simulink model "uz_pu_conversion"  (R2021a)
settings: Solver=FixedStepDiscrete  StartTime=0.0  StopTime=0.0034  RelTol=1e-3
values from neighbouring files (symbols this model uses):
  ampl = 28*sqrt(2)    [uz_pu_conversion_init.m]
  freq_Hz = 300    [uz_pu_conversion_init.m]
  I_B = sqrt(2)*I_R    [uz_pu_conversion_init.m]
  t_ADC = 1/f_ADC    (= 1e-05)    [uz_pu_conversion_init.m]
  V_B = sqrt(2/3)*V_R    [uz_pu_conversion_init.m]
  v_dc = 565    [uz_pu_conversion_init.m]
libraries: spsThreePhaseSineGeneratorLib x3, simulink x1
settings Model: DataTypeOverride=Off  Creator=micha  LastModifiedBy=micha
settings SolverCC: AlgebraicLoopSolver=TrustRegion
settings DataIOCC: LimitDataPoints=on  SaveOutput=off  SaveTime=off
settings OptimizationCC: BlockReduction=off  ConditionallyExecuteInputs=off  DefaultParameterBehavior=Inlined  LifeSpan=inf
settings DebuggingCC: AlgebraicLoopMsg=error  SingleTaskRateTransMsg=error  AllowSymbolicDim=off  StrictBusMsg=ErrorOnBusTreatedAsVector  SFUnexpectedBacktrackingDiag=warning  SFNoUnconditionalDefaultTransitionDiag=warning  SFExecutionAtInitializationDiag=none  SFMachineParentedDataDiag=warning  ArithmeticOperatorsInVariantConditions=warning
settings HardwareCC: ProdBitPerPointer=32  ProdBitPerSizeT=32  ProdBitPerPtrDiffT=32  ProdLargestAtomicFloat=None  ProdIntDivRoundTo=Undefined  ProdEndianess=Unspecified  ProdWordSize=32  ProdHWDeviceType=ASIC/FPGA->ASIC/FPGA  ProdEqTarget=off
settings SFSimCC: SimUseLocalCustomCode=off  CustomCodeUndefinedFunction=UseInterfaceOnly
settings RTWCC: RTWUseLocalCustomCode=off
settings CodeAppCC: StateflowObjectComments=on
settings GRTTargetCC: TargetLangStandard=C89/C90 (ANSI)
settings ConfigComp: CovScope=ReferencedModels  CovMetricSettings=dw  CovSaveCumulativeToWorkspaceVar=on  CovSaveSingleToWorkspaceVar=on  CovExternalEMLEnable=off  CovSFcnEnable=off

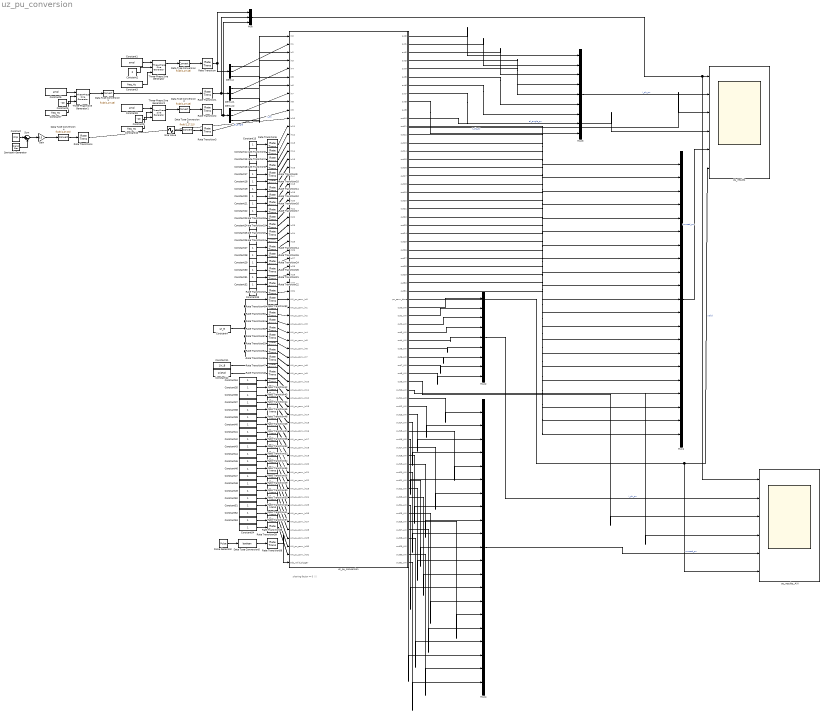
== system uz_pu_conversion ==
  note: sharing factor = 0 !!!
  Constant : Constant  Value=2*pi
  Constant1 : Constant  Value=ampl
  Constant10 : Constant  Value=freq_Hz
  Constant11 : Constant  Value=1/V_B  OutDataTypeStr=fixdt(0,18,18)
  Constant12 : Constant  Value=1/(2*pi)  OutDataTypeStr=fixdt(0,18,18)
  Constant{13..33} (21 alike) : Constant  OutDataTypeStr=fixdt(1,27,15)
  Constant2 : Constant  Value=0
  Constant3 : Constant  Value=freq_Hz
  Constant{34..54} (21 alike) : Constant  OutDataTypeStr=fixdt(0,18,18)
  Constant4 : Constant  Value=1/I_B  OutDataTypeStr=fixdt(0,18,18)
  Constant5 : Constant  Value=ampl
  Constant6 : Constant  Value=-20
  Constant7 : Constant  Value=freq_Hz
  Constant8 : Constant  Value=ampl
  Constant9 : Constant  Value=-40
  Data Type Conversion{,1..4} (5 alike) : DataTypeConversion  OutDataTypeStr=fixdt(1,27,15)
  Data Type Conversion5 : DataTypeConversion  OutDataTypeStr=boolean
  Demux : Demux  Outputs=3
  Demux1 : Demux  Outputs=3
  Demux2 : Demux  Outputs=3
  Gain : Gain  Gain=0.5
  Mux : Mux  Inputs=3
  Mux1 : Mux  Inputs=21
  Mux2 : Mux  Inputs=9
  Mux3 : Mux  Inputs=9
  Mux4 : Mux  Inputs=21
  Pulse Generator : DiscretePulseGenerator  PulseType=Time based  Period=t_ADC  PulseWidth=5
  Rate Transition{,1..58} (59 alike) : RateTransition  OutPortSampleTime=ts
  Sawtooth Generator : SignalGenerator  WaveForm=sawtooth  Amplitude=2*pi  Frequency=2*pi*freq_Hz  Units=rad/sec
  Sine Wave : Sin  Amplitude=0.03*v_dc  Bias=v_dc  Frequency=2*pi*2*9*freq_Hz  SampleTime=0
  Sum : Sum  Inputs=|+-
  Three-Phase Sine Generator : spsThreePhaseSineGeneratorLib/Three-Phase Sine Generator  Ts=10e-9
      settings: SourceProductBaseCode=PS
  Three-Phase Sine Generator1 : spsThreePhaseSineGeneratorLib/Three-Phase Sine Generator  Ts=10e-9
      settings: SourceProductBaseCode=PS
  Three-Phase Sine Generator2 : spsThreePhaseSineGeneratorLib/Three-Phase Sine Generator  Ts=10e-9
      settings: SourceProductBaseCode=PS
  pu_results : Scope  NumInputPorts=6
  pu_results_AXI : Scope  NumInputPorts=6
  uz_pu_conversion : Subsystem  TreatAsAtomicUnit=on
  wires:
  Three-Phase Sine Generator/1 -> Data Type Conversion/1
  Constant1/1 -> Three-Phase Sine Generator/1
  Constant2/1 -> Three-Phase Sine Generator/2
  Constant3/1 -> Three-Phase Sine Generator/3
  Rate Transition/1 -> Demux/1, Mux/1
  Demux/1 -> uz_pu_conversion/1(in0)
  Data Type Conversion/1 -> Rate Transition/1
  Demux/2 -> uz_pu_conversion/2(in1)
  Demux/3 -> uz_pu_conversion/3(in2)
  Constant6/1 -> Three-Phase Sine Generator1/2
  Constant7/1 -> Three-Phase Sine Generator1/3
  Data Type Conversion1/1 -> Rate Transition1/1
  Constant5/1 -> Three-Phase Sine Generator1/1
  Three-Phase Sine Generator1/1 -> Data Type Conversion1/1
  Constant4/1 -> Rate Transition56/1, Rate Transition52/1, Rate Transition49/1, Rate Transition50/1, Rate Transition51/1, Rate Transition57/1, Rate Transition53/1, Rate Transition54/1, Rate Transition55/1
  uz_pu_conversion/6(out5) -> Mux3/6
  uz_pu_conversion/5(out4) -> Mux3/5
  uz_pu_conversion/1(out0) -> Mux3/1
  uz_pu_conversion/2(out1) -> Mux3/2
  uz_pu_conversion/3(out2) -> Mux3/3
  uz_pu_conversion/4(out3) -> Mux3/4
  Mux3/1 -> pu_results/2  "i_ph_pu"
  Demux1/1 -> uz_pu_conversion/4(in3)
  Demux1/2 -> uz_pu_conversion/5(in4)
  Demux1/3 -> uz_pu_conversion/6(in5)
  Data Type Conversion2/1 -> Rate Transition2/1
  Constant8/1 -> Three-Phase Sine Generator2/1
  Three-Phase Sine Generator2/1 -> Data Type Conversion2/1
  Constant9/1 -> Three-Phase Sine Generator2/2
  Constant10/1 -> Three-Phase Sine Generator2/3
  Rate Transition2/1 -> Mux/3, Demux2/1
  Demux2/1 -> uz_pu_conversion/7(in6)
  Demux2/2 -> uz_pu_conversion/8(in7)
  Demux2/3 -> uz_pu_conversion/9(in8)
  uz_pu_conversion/7(out6) -> Mux3/7
  uz_pu_conversion/8(out7) -> Mux3/8
  uz_pu_conversion/9(out8) -> Mux3/9
  Constant11/1 -> Rate Transition47/1
  Rate Transition3/1 -> uz_pu_conversion/10(in9)  "v_dc"
  Sine Wave/1 -> Data Type Conversion3/1
  uz_pu_conversion/10(out9) -> pu_results/3  "v_dc_pu"
  Data Type Conversion3/1 -> Rate Transition3/1
  Data Type Conversion4/1 -> Rate Transition4/1
  Rate Transition4/1 -> uz_pu_conversion/11(in10)  "el_angle"
  Sawtooth Generator/1 -> Sum/2
  Constant12/1 -> Rate Transition48/1
  uz_pu_conversion/11(out10) -> pu_results/4  "el_angle_pu"
  Constant/1 -> Sum/1
  Gain/1 -> Data Type Conversion4/1
  Sum/1 -> Gain/1
  Rate Transition5/1 -> uz_pu_conversion/12(in11)
  Rate Transition6/1 -> uz_pu_conversion/13(in12)
  Rate Transition7/1 -> uz_pu_conversion/14(in13)
  Rate Transition8/1 -> uz_pu_conversion/15(in14)
  Rate Transition9/1 -> uz_pu_conversion/16(in15)
  Rate Transition10/1 -> uz_pu_conversion/17(in16)
  Rate Transition12/1 -> uz_pu_conversion/19(in18)
  Rate Transition11/1 -> uz_pu_conversion/18(in17)
  Rate Transition13/1 -> uz_pu_conversion/25(in24)
  Rate Transition16/1 -> uz_pu_conversion/20(in19)
  Rate Transition17/1 -> uz_pu_conversion/21(in20)
  Rate Transition19/1 -> uz_pu_conversion/23(in22)
  Rate Transition18/1 -> uz_pu_conversion/22(in21)
  Rate Transition20/1 -> uz_pu_conversion/24(in23)
  Rate Transition15/1 -> uz_pu_conversion/27(in26)
  Rate Transition14/1 -> uz_pu_conversion/26(in25)
  Rate Transition23/1 -> uz_pu_conversion/32(in31)
  Rate Transition22/1 -> uz_pu_conversion/31(in30)
  Rate Transition25/1 -> uz_pu_conversion/29(in28)
  Rate Transition24/1 -> uz_pu_conversion/28(in27)
  Rate Transition21/1 -> uz_pu_conversion/30(in29)
  Rate Transition34/1 -> uz_pu_conversion/54(AXI_pu_conv_in21)
  Rate Transition32/1 -> uz_pu_conversion/52(AXI_pu_conv_in19)
  Rate Transition36/1 -> uz_pu_conversion/56(AXI_pu_conv_in23)
  Rate Transition31/1 -> uz_pu_conversion/59(AXI_pu_conv_in26)
  Rate Transition43/1 -> uz_pu_conversion/45(AXI_pu_conv_in12)
  Rate Transition39/1 -> uz_pu_conversion/64(AXI_pu_conv_in31)
  Rate Transition41/1 -> uz_pu_conversion/61(AXI_pu_conv_in28)
  Rate Transition38/1 -> uz_pu_conversion/63(AXI_pu_conv_in30)
  Rate Transition30/1 -> uz_pu_conversion/58(AXI_pu_conv_in25)
  Rate Transition37/1 -> uz_pu_conversion/62(AXI_pu_conv_in29)
  Rate Transition27/1 -> uz_pu_conversion/50(AXI_pu_conv_in17)
  Rate Transition26/1 -> uz_pu_conversion/49(AXI_pu_conv_in16)
  Rate Transition40/1 -> uz_pu_conversion/60(AXI_pu_conv_in27)
  Rate Transition45/1 -> uz_pu_conversion/47(AXI_pu_conv_in14)
  Rate Transition44/1 -> uz_pu_conversion/46(AXI_pu_conv_in13)
  Rate Transition28/1 -> uz_pu_conversion/51(AXI_pu_conv_in18)
  Rate Transition35/1 -> uz_pu_conversion/55(AXI_pu_conv_in22)
  Rate Transition46/1 -> uz_pu_conversion/48(AXI_pu_conv_in15)
  Rate Transition29/1 -> uz_pu_conversion/57(AXI_pu_conv_in24)
  Rate Transition33/1 -> uz_pu_conversion/53(AXI_pu_conv_in20)
  Rate Transition42/1 -> uz_pu_conversion/44(AXI_pu_conv_in11)
  Rate Transition47/1 -> uz_pu_conversion/42(AXI_pu_conv_in9)
  Rate Transition48/1 -> uz_pu_conversion/43(AXI_pu_conv_in10)
  Rate Transition50/1 -> uz_pu_conversion/35(AXI_pu_conv_in2)
  Rate Transition49/1 -> uz_pu_conversion/34(AXI_pu_conv_in1)
  Rate Transition53/1 -> uz_pu_conversion/39(AXI_pu_conv_in6)
  Rate Transition52/1 -> uz_pu_conversion/33(AXI_pu_conv_in0)
  Rate Transition51/1 -> uz_pu_conversion/36(AXI_pu_conv_in3)
  Rate Transition54/1 -> uz_pu_conversion/40(AXI_pu_conv_in7)
  Rate Transition55/1 -> uz_pu_conversion/41(AXI_pu_conv_in8)
  Rate Transition57/1 -> uz_pu_conversion/38(AXI_pu_conv_in5)
  Rate Transition56/1 -> uz_pu_conversion/37(AXI_pu_conv_in4)
  Mux/1 -> pu_results/1, pu_results_AXI/1
  Rate Transition1/1 -> Mux/2, Demux1/1
  Constant13/1 -> Rate Transition5/1
  Constant14/1 -> Rate Transition6/1
  Constant15/1 -> Rate Transition7/1
  Constant16/1 -> Rate Transition8/1
  Constant18/1 -> Rate Transition10/1
  Constant17/1 -> Rate Transition9/1
  Constant19/1 -> Rate Transition11/1
  Constant20/1 -> Rate Transition12/1
  Constant22/1 -> Rate Transition17/1
  Constant21/1 -> Rate Transition16/1
  Constant23/1 -> Rate Transition18/1
  Constant24/1 -> Rate Transition19/1
  Constant26/1 -> Rate Transition13/1
  Constant25/1 -> Rate Transition20/1
  Constant27/1 -> Rate Transition14/1
  Constant28/1 -> Rate Transition15/1
  Constant30/1 -> Rate Transition25/1
  Constant29/1 -> Rate Transition24/1
  Constant32/1 -> Rate Transition22/1
  Constant31/1 -> Rate Transition21/1
  Constant33/1 -> Rate Transition23/1
  Constant34/1 -> Rate Transition42/1
  Constant35/1 -> Rate Transition43/1
  Constant37/1 -> Rate Transition45/1
  Constant36/1 -> Rate Transition44/1
  Constant41/1 -> Rate Transition28/1
  Constant40/1 -> Rate Transition27/1
  Constant39/1 -> Rate Transition26/1
  Constant38/1 -> Rate Transition46/1
  Constant47/1 -> Rate Transition29/1
  Constant46/1 -> Rate Transition36/1
  Constant49/1 -> Rate Transition31/1
  Constant45/1 -> Rate Transition35/1
  Constant48/1 -> Rate Transition30/1
  Constant44/1 -> Rate Transition34/1
  Constant43/1 -> Rate Transition33/1
  Constant42/1 -> Rate Transition32/1
  Constant53/1 -> Rate Transition38/1
  Constant54/1 -> Rate Transition39/1
  Constant50/1 -> Rate Transition40/1
  Constant51/1 -> Rate Transition41/1
  Constant52/1 -> Rate Transition37/1
  uz_pu_conversion/12(out11) -> Mux1/1
  uz_pu_conversion/13(out12) -> Mux1/2
  uz_pu_conversion/14(out13) -> Mux1/3
  uz_pu_conversion/15(out14) -> Mux1/4
  uz_pu_conversion/16(out15) -> Mux1/5
  uz_pu_conversion/17(out16) -> Mux1/6
  uz_pu_conversion/18(out17) -> Mux1/7
  uz_pu_conversion/19(out18) -> Mux1/8
  uz_pu_conversion/20(out19) -> Mux1/9
  uz_pu_conversion/21(out20) -> Mux1/10
  uz_pu_conversion/22(out21) -> Mux1/11
  uz_pu_conversion/23(out22) -> Mux1/12
  uz_pu_conversion/24(out23) -> Mux1/13
  uz_pu_conversion/25(out24) -> Mux1/14
  uz_pu_conversion/26(out25) -> Mux1/15
  uz_pu_conversion/27(out26) -> Mux1/16
  uz_pu_conversion/28(out27) -> Mux1/17
  uz_pu_conversion/29(out28) -> Mux1/18
  uz_pu_conversion/30(out29) -> Mux1/19
  uz_pu_conversion/31(out30) -> Mux1/20
  uz_pu_conversion/32(out31) -> Mux1/21
  Mux1/1 -> pu_results/5  "unused_pu"
  Data Type Conversion5/1 -> Rate Transition58/1
  Pulse Generator/1 -> Data Type Conversion5/1
  Rate Transition58/1 -> uz_pu_conversion/65(adc_valid_trigger)
  uz_pu_conversion/33(pu_conv_done) -> pu_results_AXI/6, pu_results/6  "valid"
  uz_pu_conversion/35(out1_AXI) -> Mux2/2
  uz_pu_conversion/34(out0_AXI) -> Mux2/1
  uz_pu_conversion/36(out2_AXI) -> Mux2/3
  uz_pu_conversion/37(out3_AXI) -> Mux2/4
  uz_pu_conversion/38(out4_AXI) -> Mux2/5
  uz_pu_conversion/39(out5_AXI) -> Mux2/6
  uz_pu_conversion/40(out6_AXI) -> Mux2/7
  uz_pu_conversion/41(out7_AXI) -> Mux2/8
  uz_pu_conversion/42(out8_AXI) -> Mux2/9
  uz_pu_conversion/45(out11_AXI) -> Mux4/1
  Mux2/1 -> pu_results_AXI/2  "i_ph_pu"
  uz_pu_conversion/43(out9_AXI) -> pu_results_AXI/3
  uz_pu_conversion/44(out10_AXI) -> pu_results_AXI/4
  uz_pu_conversion/46(out12_AXI) -> Mux4/2
  uz_pu_conversion/47(out13_AXI) -> Mux4/3
  uz_pu_conversion/48(out14_AXI) -> Mux4/4
  uz_pu_conversion/49(out15_AXI) -> Mux4/5
  uz_pu_conversion/50(out16_AXI) -> Mux4/6
  uz_pu_conversion/51(out17_AXI) -> Mux4/7
  uz_pu_conversion/52(out18_AXI) -> Mux4/8
  uz_pu_conversion/53(out19_AXI) -> Mux4/9
  uz_pu_conversion/54(out20_AXI) -> Mux4/10
  uz_pu_conversion/55(out21_AXI) -> Mux4/11
  uz_pu_conversion/56(out22_AXI) -> Mux4/12
  uz_pu_conversion/57(out23_AXI) -> Mux4/13
  uz_pu_conversion/58(out24_AXI) -> Mux4/14
  uz_pu_conversion/59(out25_AXI) -> Mux4/15
  uz_pu_conversion/60(out26_AXI) -> Mux4/16
  uz_pu_conversion/61(out27_AXI) -> Mux4/17
  uz_pu_conversion/62(out28_AXI) -> Mux4/18
  uz_pu_conversion/63(out29_AXI) -> Mux4/19
  uz_pu_conversion/64(out30_AXI) -> Mux4/20
  uz_pu_conversion/65(out31_AXI) -> Mux4/21
  Mux4/1 -> pu_results_AXI/5  "unused_pu"

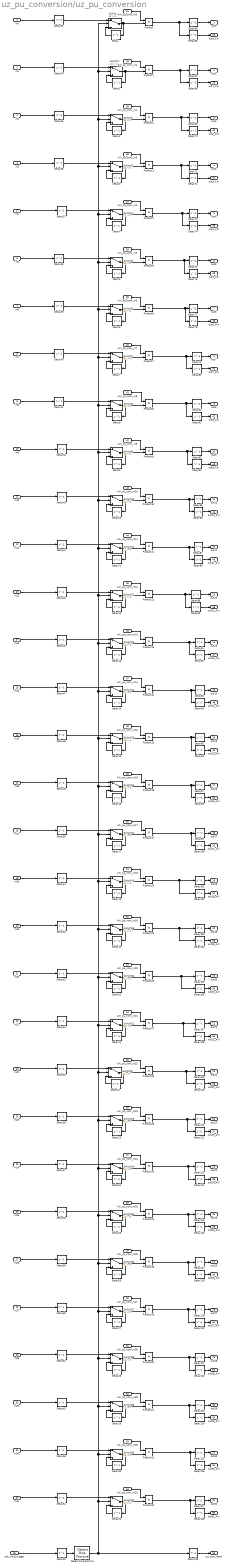
== system uz_pu_conversion/uz_pu_conversion ==
  in0 : Inport  OutDataTypeStr=fixdt(1,27,15)
  in1 : Inport  Port=2  OutDataTypeStr=fixdt(1,27,15)
  in2 : Inport  Port=3  OutDataTypeStr=fixdt(1,27,15)
  in3 : Inport  Port=4  OutDataTypeStr=fixdt(1,27,15)
  in4 : Inport  Port=5  OutDataTypeStr=fixdt(1,27,15)
  in5 : Inport  Port=6  OutDataTypeStr=fixdt(1,27,15)
  in6 : Inport  Port=7  OutDataTypeStr=fixdt(1,27,15)
  in7 : Inport  Port=8  OutDataTypeStr=fixdt(1,27,15)
  in8 : Inport  Port=9  OutDataTypeStr=fixdt(1,27,15)
  in9 : Inport  Port=10  OutDataTypeStr=fixdt(1,27,15)
  in10 : Inport  Port=11  OutDataTypeStr=fixdt(1,27,15)
  in11 : Inport  Port=12  OutDataTypeStr=fixdt(1,27,15)
  in12 : Inport  Port=13  OutDataTypeStr=fixdt(1,27,15)
  in13 : Inport  Port=14  OutDataTypeStr=fixdt(1,27,15)
  in14 : Inport  Port=15  OutDataTypeStr=fixdt(1,27,15)
  in15 : Inport  Port=16  OutDataTypeStr=fixdt(1,27,15)
  in16 : Inport  Port=17  OutDataTypeStr=fixdt(1,27,15)
  in17 : Inport  Port=18  OutDataTypeStr=fixdt(1,27,15)
  in18 : Inport  Port=19  OutDataTypeStr=fixdt(1,27,15)
  in19 : Inport  Port=20  OutDataTypeStr=fixdt(1,27,15)
  in20 : Inport  Port=21  OutDataTypeStr=fixdt(1,27,15)
  in21 : Inport  Port=22  OutDataTypeStr=fixdt(1,27,15)
  in22 : Inport  Port=23  OutDataTypeStr=fixdt(1,27,15)
  in23 : Inport  Port=24  OutDataTypeStr=fixdt(1,27,15)
  in24 : Inport  Port=25  OutDataTypeStr=fixdt(1,27,15)
  in25 : Inport  Port=26  OutDataTypeStr=fixdt(1,27,15)
  in26 : Inport  Port=27  OutDataTypeStr=fixdt(1,27,15)
  in27 : Inport  Port=28  OutDataTypeStr=fixdt(1,27,15)
  in28 : Inport  Port=29  OutDataTypeStr=fixdt(1,27,15)
  in29 : Inport  Port=30  OutDataTypeStr=fixdt(1,27,15)
  in30 : Inport  Port=31  OutDataTypeStr=fixdt(1,27,15)
  in31 : Inport  Port=32  OutDataTypeStr=fixdt(1,27,15)
  AXI_pu_conv_in0 : Inport  Port=33  OutDataTypeStr=fixdt(0,18,18)
  AXI_pu_conv_in1 : Inport  Port=34  OutDataTypeStr=fixdt(0,18,18)
  AXI_pu_conv_in2 : Inport  Port=35  OutDataTypeStr=fixdt(0,18,18)
  AXI_pu_conv_in3 : Inport  Port=36  OutDataTypeStr=fixdt(0,18,18)
  AXI_pu_conv_in4 : Inport  Port=37  OutDataTypeStr=fixdt(0,18,18)
  AXI_pu_conv_in5 : Inport  Port=38  OutDataTypeStr=fixdt(0,18,18)
  AXI_pu_conv_in6 : Inport  Port=39  OutDataTypeStr=fixdt(0,18,18)
  AXI_pu_conv_in7 : Inport  Port=40  OutDataTypeStr=fixdt(0,18,18)
  AXI_pu_conv_in8 : Inport  Port=41  OutDataTypeStr=fixdt(0,18,18)
  AXI_pu_conv_in9 : Inport  Port=42  OutDataTypeStr=fixdt(0,18,18)
  AXI_pu_conv_in10 : Inport  Port=43  OutDataTypeStr=fixdt(0,18,18)
  AXI_pu_conv_in11 : Inport  Port=44  OutDataTypeStr=fixdt(0,18,18)
  AXI_pu_conv_in12 : Inport  Port=45  OutDataTypeStr=fixdt(0,18,18)
  AXI_pu_conv_in13 : Inport  Port=46  OutDataTypeStr=fixdt(0,18,18)
  AXI_pu_conv_in14 : Inport  Port=47  OutDataTypeStr=fixdt(0,18,18)
  AXI_pu_conv_in15 : Inport  Port=48  OutDataTypeStr=fixdt(0,18,18)
  AXI_pu_conv_in16 : Inport  Port=49  OutDataTypeStr=fixdt(0,18,18)
  AXI_pu_conv_in17 : Inport  Port=50  OutDataTypeStr=fixdt(0,18,18)
  AXI_pu_conv_in18 : Inport  Port=51  OutDataTypeStr=fixdt(0,18,18)
  AXI_pu_conv_in19 : Inport  Port=52  OutDataTypeStr=fixdt(0,18,18)
  AXI_pu_conv_in20 : Inport  Port=53  OutDataTypeStr=fixdt(0,18,18)
  AXI_pu_conv_in21 : Inport  Port=54  OutDataTypeStr=fixdt(0,18,18)
  AXI_pu_conv_in22 : Inport  Port=55  OutDataTypeStr=fixdt(0,18,18)
  AXI_pu_conv_in23 : Inport  Port=56  OutDataTypeStr=fixdt(0,18,18)
  AXI_pu_conv_in24 : Inport  Port=57  OutDataTypeStr=fixdt(0,18,18)
  AXI_pu_conv_in25 : Inport  Port=58  OutDataTypeStr=fixdt(0,18,18)
  AXI_pu_conv_in26 : Inport  Port=59  OutDataTypeStr=fixdt(0,18,18)
  AXI_pu_conv_in27 : Inport  Port=60  OutDataTypeStr=fixdt(0,18,18)
  AXI_pu_conv_in28 : Inport  Port=61  OutDataTypeStr=fixdt(0,18,18)
  AXI_pu_conv_in29 : Inport  Port=62  OutDataTypeStr=fixdt(0,18,18)
  AXI_pu_conv_in30 : Inport  Port=63  OutDataTypeStr=fixdt(0,18,18)
  AXI_pu_conv_in31 : Inport  Port=64  OutDataTypeStr=fixdt(0,18,18)
  adc_valid_trigger : Inport  Port=65  OutDataTypeStr=boolean
  Delay{,1..129} (130 alike) : Delay  DelayLength=1
  Detect Rise Positive : simulink/Logic and Bit Operations/Detect Rise Positive  vinit=0  OutDataTypeStr=boolean
  Product{,1..31} (32 alike) : Product  OutDataTypeStr=pu_fixdt_type
  Switch{,1..31} (32 alike) : Switch  Criteria=u2 > Threshold
  out0 : Outport
  out1 : Outport  Port=2
  out2 : Outport  Port=3
  out3 : Outport  Port=4
  out4 : Outport  Port=5
  out5 : Outport  Port=6
  out6 : Outport  Port=7
  out7 : Outport  Port=8
  out8 : Outport  Port=9
  out9 : Outport  Port=10
  out10 : Outport  Port=11
  out11 : Outport  Port=12
  out12 : Outport  Port=13
  out13 : Outport  Port=14
  out14 : Outport  Port=15
  out15 : Outport  Port=16
  out16 : Outport  Port=17
  out17 : Outport  Port=18
  out18 : Outport  Port=19
  out19 : Outport  Port=20
  out20 : Outport  Port=21
  out21 : Outport  Port=22
  out22 : Outport  Port=23
  out23 : Outport  Port=24
  out24 : Outport  Port=25
  out25 : Outport  Port=26
  out26 : Outport  Port=27
  out27 : Outport  Port=28
  out28 : Outport  Port=29
  out29 : Outport  Port=30
  out30 : Outport  Port=31
  out31 : Outport  Port=32
  pu_conv_done : Outport  Port=33  OutDataTypeStr=boolean  LockScale=on
  out0_AXI : Outport  Port=34
  out1_AXI : Outport  Port=35
  out2_AXI : Outport  Port=36
  out3_AXI : Outport  Port=37
  out4_AXI : Outport  Port=38
  out5_AXI : Outport  Port=39
  out6_AXI : Outport  Port=40
  out7_AXI : Outport  Port=41
  out8_AXI : Outport  Port=42
  out9_AXI : Outport  Port=43
  out10_AXI : Outport  Port=44
  out11_AXI : Outport  Port=45
  out12_AXI : Outport  Port=46
  out13_AXI : Outport  Port=47
  out14_AXI : Outport  Port=48
  out15_AXI : Outport  Port=49
  out16_AXI : Outport  Port=50
  out17_AXI : Outport  Port=51
  out18_AXI : Outport  Port=52
  out19_AXI : Outport  Port=53
  out20_AXI : Outport  Port=54
  out21_AXI : Outport  Port=55
  out22_AXI : Outport  Port=56
  out23_AXI : Outport  Port=57
  out24_AXI : Outport  Port=58
  out25_AXI : Outport  Port=59
  out26_AXI : Outport  Port=60
  out27_AXI : Outport  Port=61
  out28_AXI : Outport  Port=62
  out29_AXI : Outport  Port=63
  out30_AXI : Outport  Port=64
  out31_AXI : Outport  Port=65
  wires:
  AXI_pu_conv_in0/1 -> Product/1
  Product/1 -> Delay65/1, Delay66/1
  AXI_pu_conv_in1/1 -> Product1/1
  Product1/1 -> Delay67/1, Delay68/1
  AXI_pu_conv_in2/1 -> Product2/1
  Product3/1 -> Delay71/1, Delay72/1
  Product2/1 -> Delay69/1, Delay70/1
  AXI_pu_conv_in3/1 -> Product3/1
  AXI_pu_conv_in4/1 -> Product4/1
  AXI_pu_conv_in7/1 -> Product7/1
  Product7/1 -> Delay79/1, Delay80/1
  Product6/1 -> Delay77/1, Delay78/1
  Product5/1 -> Delay75/1, Delay76/1
  AXI_pu_conv_in6/1 -> Product6/1
  Product4/1 -> Delay73/1, Delay74/1
  AXI_pu_conv_in5/1 -> Product5/1
  AXI_pu_conv_in8/1 -> Product8/1
  AXI_pu_conv_in11/1 -> Product11/1
  Product10/1 -> Delay85/1, Delay86/1
  Product11/1 -> Delay87/1, Delay88/1
  AXI_pu_conv_in10/1 -> Product10/1
  AXI_pu_conv_in9/1 -> Product9/1
  AXI_pu_conv_in14/1 -> Product14/1
  Product12/1 -> Delay89/1, Delay90/1
  AXI_pu_conv_in13/1 -> Product13/1
  AXI_pu_conv_in15/1 -> Product15/1
  Product9/1 -> Delay83/1, Delay84/1
  Product14/1 -> Delay93/1, Delay94/1
  Product13/1 -> Delay91/1, Delay92/1
  Product8/1 -> Delay81/1, Delay82/1
  AXI_pu_conv_in12/1 -> Product12/1
  Product15/1 -> Delay95/1, Delay96/1
  Product30/1 -> Delay113/1, Delay114/1
  Product23/1 -> Delay127/1, Delay128/1
  AXI_pu_conv_in28/1 -> Product20/1
  AXI_pu_conv_in29/1 -> Product21/1
  Product20/1 -> Delay121/1, Delay122/1
  Product31/1 -> Delay115/1, Delay116/1
  AXI_pu_conv_in25/1 -> Product31/1
  AXI_pu_conv_in24/1 -> Product30/1
  Product18/1 -> Delay117/1, Delay118/1
  AXI_pu_conv_in27/1 -> Product19/1
  Product19/1 -> Delay119/1, Delay120/1
  AXI_pu_conv_in31/1 -> Product23/1
  AXI_pu_conv_in16/1 -> Product16/1
  AXI_pu_conv_in26/1 -> Product18/1
  AXI_pu_conv_in19/1 -> Product25/1
  Product24/1 -> Delay101/1, Delay102/1
  Product25/1 -> Delay103/1, Delay104/1
  AXI_pu_conv_in18/1 -> Product24/1
  AXI_pu_conv_in17/1 -> Product17/1
  AXI_pu_conv_in22/1 -> Product28/1
  AXI_pu_conv_in30/1 -> Product22/1
  Product26/1 -> Delay105/1, Delay106/1
  AXI_pu_conv_in21/1 -> Product27/1
  AXI_pu_conv_in23/1 -> Product29/1
  Product17/1 -> Delay99/1, Delay100/1
  Product28/1 -> Delay109/1, Delay110/1
  Product27/1 -> Delay107/1, Delay108/1
  Product21/1 -> Delay123/1, Delay124/1
  Product16/1 -> Delay97/1, Delay98/1
  AXI_pu_conv_in20/1 -> Product26/1
  Product29/1 -> Delay111/1, Delay112/1
  Switch/1 -> Product/2, Delay/1
  Delay/1 -> Switch/3
  Switch1/1 -> Product1/2, Delay1/1
  Delay1/1 -> Switch1/3
  Switch2/1 -> Product2/2, Delay2/1
  Delay2/1 -> Switch2/3
  Switch3/1 -> Product3/2, Delay3/1
  Delay3/1 -> Switch3/3
  Switch4/1 -> Product4/2, Delay4/1
  Delay4/1 -> Switch4/3
  Switch5/1 -> Product5/2, Delay5/1
  Delay5/1 -> Switch5/3
  Switch6/1 -> Product6/2, Delay6/1
  Delay6/1 -> Switch6/3
  Switch7/1 -> Product7/2, Delay7/1
  Delay7/1 -> Switch7/3
  Switch8/1 -> Product8/2, Delay8/1
  Delay8/1 -> Switch8/3
  Switch9/1 -> Product9/2, Delay9/1
  Delay9/1 -> Switch9/3
  Switch10/1 -> Product10/2, Delay10/1
  Delay10/1 -> Switch10/3
  Switch11/1 -> Product11/2, Delay11/1
  Delay11/1 -> Switch11/3
  Switch12/1 -> Product12/2, Delay12/1
  Delay12/1 -> Switch12/3
  Switch13/1 -> Product13/2, Delay13/1
  Delay13/1 -> Switch13/3
  Switch14/1 -> Product14/2, Delay14/1
  Delay14/1 -> Switch14/3
  Switch15/1 -> Product15/2, Delay15/1
  Delay15/1 -> Switch15/3
  Switch16/1 -> Product16/2, Delay16/1
  Delay16/1 -> Switch16/3
  Switch17/1 -> Product17/2, Delay17/1
  Delay17/1 -> Switch17/3
  Switch18/1 -> Product24/2, Delay18/1
  Delay18/1 -> Switch18/3
  Switch19/1 -> Product25/2, Delay19/1
  Delay19/1 -> Switch19/3
  Switch20/1 -> Product26/2, Delay20/1
  Delay20/1 -> Switch20/3
  Switch21/1 -> Product27/2, Delay21/1
  Delay21/1 -> Switch21/3
  Switch22/1 -> Product28/2, Delay22/1
  Delay22/1 -> Switch22/3
  Switch23/1 -> Product29/2, Delay23/1
  Delay23/1 -> Switch23/3
  Switch24/1 -> Product30/2, Delay24/1
  Delay24/1 -> Switch24/3
  Switch25/1 -> Product31/2, Delay25/1
  Delay25/1 -> Switch25/3
  Switch26/1 -> Product18/2, Delay26/1
  Delay26/1 -> Switch26/3
  Switch27/1 -> Product19/2, Delay27/1
  Delay27/1 -> Switch27/3
  Switch28/1 -> Product20/2, Delay28/1
  Delay28/1 -> Switch28/3
  Switch29/1 -> Product21/2, Delay29/1
  Delay29/1 -> Switch29/3
  Switch30/1 -> Product22/2, Delay30/1
  Delay30/1 -> Switch30/3
  Switch31/1 -> Product23/2, Delay31/1
  Delay31/1 -> Switch31/3
  Detect Rise Positive/1 -> Delay129/1, Switch31/2, Switch30/2, Switch29/2, Switch28/2, Switch27/2, Switch26/2, Switch25/2, Switch24/2, Switch23/2, Switch22/2, Switch21/2, Switch20/2, Switch19/2, Switch18/2, Switch17/2, Switch16/2, Switch15/2, Switch14/2, Switch13/2, Switch11/2, Switch10/2, Switch9/2, Switch7/2, Switch6/2, Switch5/2, Switch3/2, Switch2/2, Switch1/2, Switch/2, Switch4/2, Switch8/2, Switch12/2
  adc_valid_trigger/1 -> Delay32/1
  Product22/1 -> Delay125/1, Delay126/1
  Delay32/1 -> Detect Rise Positive/1
  in0/1 -> Delay33/1
  Delay33/1 -> Switch/1
  in1/1 -> Delay34/1
  Delay34/1 -> Switch1/1
  in2/1 -> Delay35/1
  Delay35/1 -> Switch2/1
  in3/1 -> Delay36/1
  Delay36/1 -> Switch3/1
  in4/1 -> Delay37/1
  Delay37/1 -> Switch4/1
  in5/1 -> Delay38/1
  Delay38/1 -> Switch5/1
  in6/1 -> Delay39/1
  Delay39/1 -> Switch6/1
  in7/1 -> Delay40/1
  Delay40/1 -> Switch7/1
  in8/1 -> Delay41/1
  Delay41/1 -> Switch8/1
  in9/1 -> Delay42/1
  Delay42/1 -> Switch9/1
  in10/1 -> Delay43/1
  Delay43/1 -> Switch10/1
  in11/1 -> Delay44/1
  Delay44/1 -> Switch11/1
  in12/1 -> Delay45/1
  Delay45/1 -> Switch12/1
  in13/1 -> Delay46/1
  Delay46/1 -> Switch13/1
  in14/1 -> Delay47/1
  Delay47/1 -> Switch14/1
  in15/1 -> Delay48/1
  Delay48/1 -> Switch15/1
  in16/1 -> Delay49/1
  Delay49/1 -> Switch16/1
  in17/1 -> Delay50/1
  Delay50/1 -> Switch17/1
  in18/1 -> Delay51/1
  Delay51/1 -> Switch18/1
  in19/1 -> Delay52/1
  Delay52/1 -> Switch19/1
  in20/1 -> Delay53/1
  Delay53/1 -> Switch20/1
  in21/1 -> Delay54/1
  Delay54/1 -> Switch21/1
  in22/1 -> Delay55/1
  Delay55/1 -> Switch22/1
  in23/1 -> Delay56/1
  Delay56/1 -> Switch23/1
  in24/1 -> Delay57/1
  Delay57/1 -> Switch24/1
  in25/1 -> Delay58/1
  Delay58/1 -> Switch25/1
  in26/1 -> Delay59/1
  Delay59/1 -> Switch26/1
  in27/1 -> Delay60/1
  Delay60/1 -> Switch27/1
  in28/1 -> Delay61/1
  Delay61/1 -> Switch28/1
  in29/1 -> Delay62/1
  Delay62/1 -> Switch29/1
  in30/1 -> Delay63/1
  Delay63/1 -> Switch30/1
  in31/1 -> Delay64/1
  Delay64/1 -> Switch31/1
  Delay65/1 -> out0/1
  Delay66/1 -> out0_AXI/1
  Delay67/1 -> out1/1
  Delay68/1 -> out1_AXI/1
  Delay69/1 -> out2/1
  Delay70/1 -> out2_AXI/1
  Delay71/1 -> out3/1
  Delay72/1 -> out3_AXI/1
  Delay73/1 -> out4/1
  Delay74/1 -> out4_AXI/1
  Delay75/1 -> out5/1
  Delay76/1 -> out5_AXI/1
  Delay77/1 -> out6/1
  Delay78/1 -> out6_AXI/1
  Delay79/1 -> out7/1
  Delay80/1 -> out7_AXI/1
  Delay81/1 -> out8/1
  Delay82/1 -> out8_AXI/1
  Delay83/1 -> out9/1
  Delay84/1 -> out9_AXI/1
  Delay85/1 -> out10/1
  Delay86/1 -> out10_AXI/1
  Delay87/1 -> out11/1
  Delay88/1 -> out11_AXI/1
  Delay89/1 -> out12/1
  Delay90/1 -> out12_AXI/1
  Delay91/1 -> out13/1
  Delay92/1 -> out13_AXI/1
  Delay93/1 -> out14/1
  Delay94/1 -> out14_AXI/1
  Delay95/1 -> out15/1
  Delay96/1 -> out15_AXI/1
  Delay97/1 -> out16/1
  Delay98/1 -> out16_AXI/1
  Delay99/1 -> out17/1
  Delay100/1 -> out17_AXI/1
  Delay101/1 -> out18/1
  Delay102/1 -> out18_AXI/1
  Delay103/1 -> out19/1
  Delay104/1 -> out19_AXI/1
  Delay105/1 -> out20/1
  Delay106/1 -> out20_AXI/1
  Delay107/1 -> out21/1
  Delay108/1 -> out21_AXI/1
  Delay109/1 -> out22/1
  Delay110/1 -> out22_AXI/1
  Delay111/1 -> out23/1
  Delay112/1 -> out23_AXI/1
  Delay113/1 -> out24/1
  Delay114/1 -> out24_AXI/1
  Delay115/1 -> out25/1
  Delay116/1 -> out25_AXI/1
  Delay117/1 -> out26/1
  Delay118/1 -> out26_AXI/1
  Delay119/1 -> out27/1
  Delay120/1 -> out27_AXI/1
  Delay121/1 -> out28/1
  Delay122/1 -> out28_AXI/1
  Delay123/1 -> out29/1
  Delay124/1 -> out29_AXI/1
  Delay125/1 -> out30/1
  Delay126/1 -> out30_AXI/1
  Delay127/1 -> out31/1
  Delay128/1 -> out31_AXI/1
  Delay129/1 -> pu_conv_done/1
